simulink model "test_mysys"  (R2019a)
settings: Solver=VariableStepAuto  StartTime=0.0  StopTime=simTime  RelTol=1e-3
values from neighbouring files (symbols this model uses):
  delta = 1    [tset_1.m]
  den = [1 1]    [tset_1.m]
  num = [1]    [tset_1.m]
settings Model: Creator=lzr96  LastModifiedBy=lzr96
settings DataIOCC: ReturnWorkspaceOutputs=off

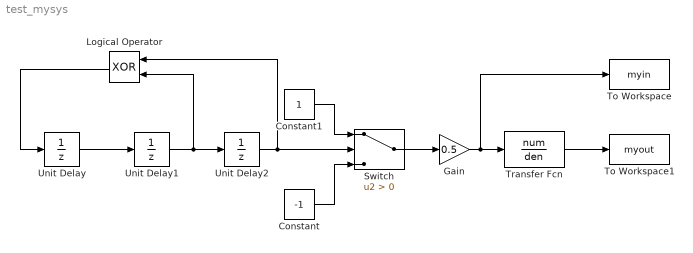
== system test_mysys ==
  Constant : Constant  Value=-1
  Constant1 : Constant
  Gain : Gain  Gain=0.5
  Logical Operator : Logic  Operator=XOR  AllPortsSameDT=off  OutDataTypeStr=boolean
  Switch : Switch  Criteria=u2 > Threshold
  To Workspace : ToWorkspace  VariableName=myin  SampleTime=delta
  To Workspace1 : ToWorkspace  VariableName=myout  SampleTime=delta
  Transfer Fcn : TransferFcn  Numerator=num  Denominator=den
  Unit Delay : UnitDelay  SampleTime=delta  HasFrameUpgradeWarning=on
  Unit Delay1 : UnitDelay  InitialCondition=1  SampleTime=delta  HasFrameUpgradeWarning=on
  Unit Delay2 : UnitDelay  SampleTime=delta  HasFrameUpgradeWarning=on
  wires:
  Unit Delay/1 -> Unit Delay1/1
  Unit Delay1/1 -> Logical Operator/2, Unit Delay2/1
  Unit Delay2/1 -> Logical Operator/1, Switch/2
  Constant/1 -> Switch/3
  Constant1/1 -> Switch/1
  Switch/1 -> Gain/1
  Logical Operator/1 -> Unit Delay/1
  Gain/1 -> To Workspace/1, Transfer Fcn/1
  Transfer Fcn/1 -> To Workspace1/1
